simulink model "Problem_2"  (R2020a)
settings: Solver=VariableStepAuto  StartTime=0.0  StopTime=10  RelTol=1e-3
undefined symbols (not defined in the file): GREEN, RED, YELLOW
settings Model: Creator=Saqlain  LastModifiedBy=Saqlain

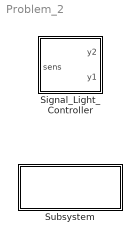
== system Problem_2 ==
  Signal_Light_Controller : Stateflow chart  TreatAsAtomicUnit=on
  Subsystem : Subsystem

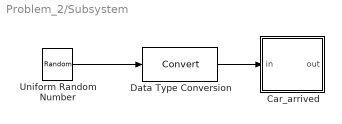
== system Problem_2/Subsystem ==
  Car_arrived : Stateflow chart  TreatAsAtomicUnit=on
  Data Type Conversion : DataTypeConversion
  Uniform Random Number : UniformRandomNumber  Minimum=0  Maximum=100  Seed=177836  SampleTime=0
  wires:
  Uniform Random Number/1 -> Data Type Conversion/1
  Data Type Conversion/1 -> Car_arrived/1(in)

== stateflow chart Problem_2/Signal_Light_Controller ==
  state StartForTraffic
    y1 = RED;
    y2 = GREEN;
  state Stop
    y1 = RED;
    y2 = GREEN;
  state StopForTraffic
    y1 = RED;
    y2 = GREEN;
  state GoToStop
    y1 = YELLOW;
    y2 = RED;
  state Go
    y1 = GREEN;
    y2 = RED;
  (default) -> Stop
  Stop -> StopForTraffic : after(20,tick)
  StopForTraffic -> StartForTraffic : [sens]
  StartForTraffic -> Go : after(3,tick)
  GoToStop -> Stop : after(3,tick)
  Go -> GoToStop : after(10,tick)
  data: sens input; y2 output; y1 output; GREEN parameter; RED parameter; YELLOW parameter

== stateflow chart Problem_2/Subsystem/Car_arrived ==
  (default) -> (junction 2) : {out = in > 98;}
  data: in input int8; out output double
